simulink model "InvPendSim"  (R2019a)
settings: Solver=ode45  StartTime=0.0  StopTime=10  RelTol=1e-3  EnableMultiTasking=on
values from neighbouring files (symbols this model uses):
  ref = -1    [NonLinearSim.m]
  ref2 = -1    [NonLinearSim.m]
libraries: cstblocks x2, dspsrcs4 x1, simulink_extras x1
settings Model: Creator=FawaD KhaN  LastModifiedBy=FawadFarooq
settings DataIOCC: LimitDataPoints=on  SaveFormat=Array  ReturnWorkspaceOutputs=off
settings OptimizationCC: LifeSpan=inf
settings DebuggingCC: SFUnexpectedBacktrackingDiag=warning  SFNoUnconditionalDefaultTransitionDiag=warning  SFExecutionAtInitializationDiag=none  ArithmeticOperatorsInVariantConditions=warning
settings HardwareCC: ProdBitPerPointer=32  ProdBitPerSizeT=32  ProdBitPerPtrDiffT=32  ProdLargestAtomicFloat=None  ProdIntDivRoundTo=Undefined  ProdEndianess=Unspecified  ProdWordSize=32  ProdHWDeviceType=32-bit Generic
settings ModelReferenceCC: PropagateSignalLabelsOutOfModel=off
settings SFSimCC: SimUseLocalCustomCode=off
settings RTWCC: RTWUseLocalCustomCode=off
settings CodeAppCC: StateflowObjectComments=on
settings GRTTargetCC: TargetLangStandard=C89/C90 (ANSI)  GeneratePreprocessorConditionals=Disable all
settings ConfigComp: CovMetricSettings=dw  CovHtmlReporting=on  CovSaveCumulativeToWorkspaceVar=on  CovSaveSingleToWorkspaceVar=on  CovExternalEMLEnable=off

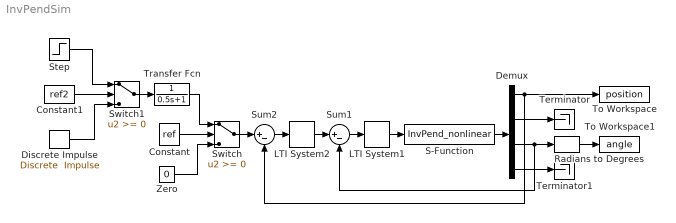
== system InvPendSim ==
  Constant : Constant  Value=ref
  Constant1 : Constant  Value=ref2
  Demux : Demux
  Discrete Impulse : dspsrcs4/Discrete  Impulse  Delay=0  SampleTime=1  FrameSample=1  OutputFrames=off  dataType=double  isSigned=on  wordLen=16  udDataType=sfix(16)  fracBitsMode=Best precision  numFracBits=15  OutDataTypeStr=double  LastOutDataTypeStr=double
  LTI System1 : cstblocks/LTI System  sys=Kth  IC=[]
  LTI System2 : cstblocks/LTI System  sys=Kx  IC=[]
  Radians to Degrees : simulink_extras/Transformations/Radians to Degrees
  S-Function : S-Function  FunctionName=InvPend_nonlinear  Parameters=x0  SFunctionDeploymentMode=off  EnableBusSupport=off
  Step : Step  Time=0.1  SampleTime=0
  Sum1 : Sum  Inputs=|+-
  Sum2 : Sum  Inputs=|+-
  Switch : Switch
  Switch1 : Switch
  Terminator : Terminator
  Terminator1 : Terminator
  To Workspace : ToWorkspace  VariableName=position  SaveFormat=Timeseries  SampleTime=-1
  To Workspace1 : ToWorkspace  VariableName=angle  SaveFormat=Timeseries  SampleTime=-1
  Transfer Fcn : TransferFcn  Denominator=[0.5 1]
  Zero : Constant  Value=0  OutDataTypeStr=Inherit: Inherit via back propagation
  wires:
  Radians to Degrees/1 -> To Workspace1/1
  LTI System1/1 -> S-Function/1
  Sum1/1 -> LTI System1/1
  Demux/3 -> Radians to Degrees/1, Sum1/2
  Demux/1 -> To Workspace/1, Sum2/2
  Demux/2 -> Terminator/1
  Demux/4 -> Terminator1/1
  S-Function/1 -> Demux/1
  Sum2/1 -> LTI System2/1
  LTI System2/1 -> Sum1/1
  Step/1 -> Switch1/1
  Transfer Fcn/1 -> Switch/1
  Zero/1 -> Switch/3
  Constant/1 -> Switch/2
  Switch/1 -> Sum2/1
  Switch1/1 -> Transfer Fcn/1
  Constant1/1 -> Switch1/2
  Discrete Impulse/1 -> Switch1/3
